simulink model "Regler_Block"  (Simulink 7.5)
settings: Solver=ode45  StartTime=0.0  StopTime=10.0  RelTol=1e-3
values from neighbouring files (symbols this model uses):
  K_ret = place(System.a, System.b, [-18 -10 -9 -5 -7])    [Test_Reglerauslegung.m]    (also in auslegung.m = place(System.a, System.b, [-2 -4 -3]))
  KV = KV'    [Reglerauslegung.m]    (also in Test_Reglerauslegung.m; auslegung.m)
undefined symbols (not defined in the file or in its folder): Control_lib, PID_Regler, Ts
libraries: simulink x8
settings Model: Creator=Mattse  LastModifiedBy=Mattse

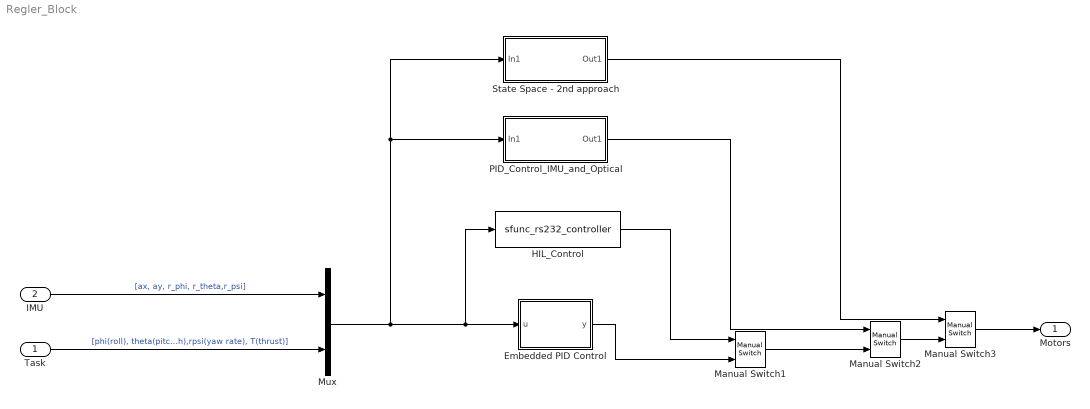
== system Regler_Block ==
  Task : Inport  PortDimensions=4  DataType=double  OutDataTypeStr=double
  IMU : Inport  Port=2
  Embedded PID Control : Stateflow chart  TreatAsAtomicUnit=on
  HIL_Control : S-Function  FunctionName=sfunc_rs232_controller  Parameters=Config  EnableBusSupport=off  mask{enabled=off}
      mask prompts: enabled "Enable this Block:"
      mask init:
      | Config.Enabled = enabled;
  Manual Switch1 : simulink/Signal Routing/Manual Switch  SystemSampleTime=-1  sw=1  action=0  varsize=off
  Manual Switch2 : simulink/Signal Routing/Manual Switch  SystemSampleTime=-1  sw=0  action=0  varsize=off
  Manual Switch3 : simulink/Signal Routing/Manual Switch  SystemSampleTime=-1  sw=1  action=0  varsize=off
  Mux : Mux  Inputs=2
  PID_Control_IMU_and_Optical : Subsystem  AncestorBlock=Control_lib/PID_Regler
  State Space - 2nd approach : Subsystem
  Motors : Outport  PortDimensions=4
  wires:
  IMU/1 -> Mux/1  "[ax, ay, r_phi, r_theta,r_psi]"
  Task/1 -> Mux/2  "[phi(roll), theta(pitch),rpsi(yaw rate), T(thrust)]"
  Mux/1 -> PID_Control_IMU_and_Optical/1(In1), State Space - 2nd approach/1(In1), HIL_Control/1, Embedded PID Control/1(u)
  Manual Switch1/1 -> Manual Switch2/2
  Embedded PID Control/1(y) -> Manual Switch1/2
  HIL_Control/1 -> Manual Switch1/1
  PID_Control_IMU_and_Optical/1(Out1) -> Manual Switch2/1
  Manual Switch2/1 -> Manual Switch3/2
  Manual Switch3/1 -> Motors/1
  State Space - 2nd approach/1(Out1) -> Manual Switch3/1

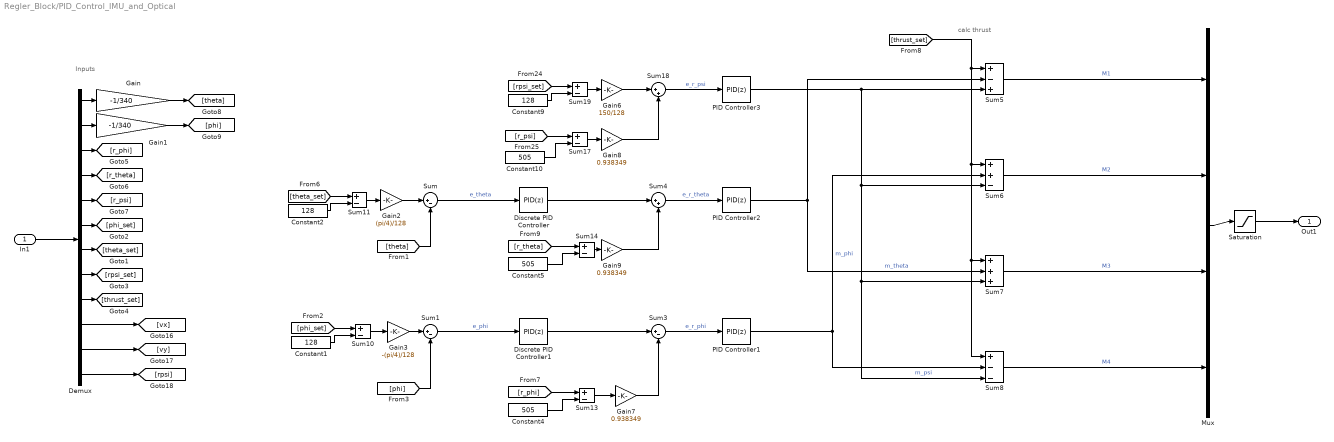
== system Regler_Block/PID_Control_IMU_and_Optical ==
  note: calc thrust
  note: Inputs
  In1 : Inport  OutDataType=fixdt(1, 16)  OutScaling=2^0
  Constant1 : Constant  Value=128  OutDataType=fixdt(1, 16)  OutScaling=2^0
  Constant10 : Constant  Value=505  OutDataType=fixdt(1, 16)  OutScaling=2^0
  Constant2 : Constant  Value=128  OutDataType=fixdt(1, 16)  OutScaling=2^0
  Constant4 : Constant  Value=505  OutDataType=fixdt(1, 16)  OutScaling=2^0
  Constant5 : Constant  Value=505  OutDataType=fixdt(1, 16)  OutScaling=2^0
  Constant9 : Constant  Value=128  OutDataType=fixdt(1, 16)  OutScaling=2^0
  Demux : Demux  Outputs=12
  Discrete PID Controller : simulink/Continuous/PID Controller  DialogController=pidpack.PIDConfig.pidDDGCreate  DialogControllerArgs=DataTag0  SystemSampleTime=-1  Controller=PID  TimeDomain=Discrete-time  SampleTime=Ts  IntegratorMethod=Forward Euler  FilterMethod=Forward Euler  Form=Ideal  P=150  I=0.5  D=0  N=0  InitialConditionSource=internal  InitialConditionForIntegrator=0  InitialConditionForFilter=0  ExternalReset=none  ZeroCross=off  LimitOutput=off  UpperSaturationLimit=inf  LowerSaturationLimit=-inf  LinearizeAsGain=off  AntiWindupMode=none  Kb=1  TrackingMode=off  Kt=1  PParamMin=[]  PParamMax=[]  IParamMin=[]  IParamMax=[]  DParamMin=[]  DParamMax=[]  NParamMin=[]  NParamMax=[]  KbParamMin=[]  KbParamMax=[]  KtParamMin=[]  KtParamMax=[]  POutMin=[]  POutMax=[]  IOutMin=[]  IOutMax=[]  DOutMin=[]  DOutMax=[]  NOutMin=[]  NOutMax=[]  KbOutMin=[]  KbOutMax=[]  KtOutMin=[]  KtOutMax=[]  IntegratorOutMin=[]  IntegratorOutMax=[]  FilterOutMin=[]  FilterOutMax=[]  SumOutMin=[]  SumOutMax=[]  SumI1OutMin=[]  SumI1OutMax=[]  SumI2OutMin=[]  SumI2OutMax=[]  SumI3OutMin=[]  SumI3OutMax=[]  SumDOutMin=[]  SumDOutMax=[]  SaturationOutMin=[]  SaturationOutMax=[]  IntegratorContinuousStateAttributes=''  IntegratorStateMustResolveToSignalObject=off  IntegratorRTWStateStorageClass=Auto  FilterContinuousStateAttributes=''  FilterStateMustResolveToSignalObject=off  FilterRTWStateStorageClass=Auto
  Discrete PID Controller1 : simulink/Continuous/PID Controller  DialogController=pidpack.PIDConfig.pidDDGCreate  DialogControllerArgs=DataTag1  SystemSampleTime=-1  Controller=PID  TimeDomain=Discrete-time  SampleTime=Ts  IntegratorMethod=Forward Euler  FilterMethod=Forward Euler  Form=Ideal  P=150  I=0.5  D=0  N=0  InitialConditionSource=internal  InitialConditionForIntegrator=0  InitialConditionForFilter=0  ExternalReset=none  ZeroCross=off  LimitOutput=off  UpperSaturationLimit=inf  LowerSaturationLimit=-inf  LinearizeAsGain=off  AntiWindupMode=none  Kb=1  TrackingMode=off  Kt=1  PParamMin=[]  PParamMax=[]  IParamMin=[]  IParamMax=[]  DParamMin=[]  DParamMax=[]  NParamMin=[]  NParamMax=[]  KbParamMin=[]  KbParamMax=[]  KtParamMin=[]  KtParamMax=[]  POutMin=[]  POutMax=[]  IOutMin=[]  IOutMax=[]  DOutMin=[]  DOutMax=[]  NOutMin=[]  NOutMax=[]  KbOutMin=[]  KbOutMax=[]  KtOutMin=[]  KtOutMax=[]  IntegratorOutMin=[]  IntegratorOutMax=[]  FilterOutMin=[]  FilterOutMax=[]  SumOutMin=[]  SumOutMax=[]  SumI1OutMin=[]  SumI1OutMax=[]  SumI2OutMin=[]  SumI2OutMax=[]  SumI3OutMin=[]  SumI3OutMax=[]  SumDOutMin=[]  SumDOutMax=[]  SaturationOutMin=[]  SaturationOutMax=[]  IntegratorContinuousStateAttributes=''  IntegratorStateMustResolveToSignalObject=off  IntegratorRTWStateStorageClass=Auto  FilterContinuousStateAttributes=''  FilterStateMustResolveToSignalObject=off  FilterRTWStateStorageClass=Auto
  Gain : Gain  Gain=-1/340  ParameterDataType=fixdt(1, 16)  ParameterScaling=2^0  OutDataType=fixdt(1, 16)  OutScaling=2^0
  Gain1 : Gain  Gain=-1/340  ParameterDataType=fixdt(1, 16)  ParameterScaling=2^0  OutDataType=fixdt(1, 16)  OutScaling=2^0
  Gain2 : Gain  Gain=(pi/4)/128  ParameterDataType=fixdt(1, 16)  ParameterScaling=2^0  OutDataType=fixdt(1, 16)  OutScaling=2^0
  Gain3 : Gain  Gain=-(pi/4)/128  ParameterDataType=fixdt(1, 16)  ParameterScaling=2^0  OutDataType=fixdt(1, 16)  OutScaling=2^0
  Gain6 : Gain  Gain=150/128  ParameterDataType=fixdt(1, 16)  ParameterScaling=2^0  OutDataType=fixdt(1, 16)  OutScaling=2^0
  Gain7 : Gain  Gain=0.938349  ParameterDataType=fixdt(1, 16)  ParameterScaling=2^0  OutDataType=fixdt(1, 16)  OutScaling=2^0
  Gain8 : Gain  Gain=0.938349  ParameterDataType=fixdt(1, 16)  ParameterScaling=2^0  OutDataType=fixdt(1, 16)  OutScaling=2^0
  Gain9 : Gain  Gain=0.938349  ParameterDataType=fixdt(1, 16)  ParameterScaling=2^0  OutDataType=fixdt(1, 16)  OutScaling=2^0
  Mux : Mux
  PID Controller1 : simulink/Continuous/PID Controller  DialogController=pidpack.PIDConfig.pidDDGCreate  DialogControllerArgs=DataTag2  SystemSampleTime=-1  Controller=PID  TimeDomain=Discrete-time  SampleTime=Ts  IntegratorMethod=Forward Euler  FilterMethod=Forward Euler  Form=Ideal  P=60  I=0.5  D=0  N=0  InitialConditionSource=internal  InitialConditionForIntegrator=0  InitialConditionForFilter=0  ExternalReset=none  ZeroCross=off  LimitOutput=off  UpperSaturationLimit=inf  LowerSaturationLimit=-inf  LinearizeAsGain=off  AntiWindupMode=none  Kb=1  TrackingMode=off  Kt=1  PParamMin=[]  PParamMax=[]  IParamMin=[]  IParamMax=[]  DParamMin=[]  DParamMax=[]  NParamMin=[]  NParamMax=[]  KbParamMin=[]  KbParamMax=[]  KtParamMin=[]  KtParamMax=[]  POutMin=[]  POutMax=[]  IOutMin=[]  IOutMax=[]  DOutMin=[]  DOutMax=[]  NOutMin=[]  NOutMax=[]  KbOutMin=[]  KbOutMax=[]  KtOutMin=[]  KtOutMax=[]  IntegratorOutMin=[]  IntegratorOutMax=[]  FilterOutMin=[]  FilterOutMax=[]  SumOutMin=[]  SumOutMax=[]  SumI1OutMin=[]  SumI1OutMax=[]  SumI2OutMin=[]  SumI2OutMax=[]  SumI3OutMin=[]  SumI3OutMax=[]  SumDOutMin=[]  SumDOutMax=[]  SaturationOutMin=[]  SaturationOutMax=[]  IntegratorContinuousStateAttributes=''  IntegratorStateMustResolveToSignalObject=off  IntegratorRTWStateStorageClass=Auto  FilterContinuousStateAttributes=''  FilterStateMustResolveToSignalObject=off  FilterRTWStateStorageClass=Auto
  PID Controller2 : simulink/Continuous/PID Controller  DialogController=pidpack.PIDConfig.pidDDGCreate  DialogControllerArgs=DataTag3  SystemSampleTime=-1  Controller=PID  TimeDomain=Discrete-time  SampleTime=Ts  IntegratorMethod=Forward Euler  FilterMethod=Forward Euler  Form=Ideal  P=60  I=0.5  D=0  N=0  InitialConditionSource=internal  InitialConditionForIntegrator=0  InitialConditionForFilter=0  ExternalReset=none  ZeroCross=off  LimitOutput=off  UpperSaturationLimit=inf  LowerSaturationLimit=-inf  LinearizeAsGain=off  AntiWindupMode=none  Kb=1  TrackingMode=off  Kt=1  PParamMin=[]  PParamMax=[]  IParamMin=[]  IParamMax=[]  DParamMin=[]  DParamMax=[]  NParamMin=[]  NParamMax=[]  KbParamMin=[]  KbParamMax=[]  KtParamMin=[]  KtParamMax=[]  POutMin=[]  POutMax=[]  IOutMin=[]  IOutMax=[]  DOutMin=[]  DOutMax=[]  NOutMin=[]  NOutMax=[]  KbOutMin=[]  KbOutMax=[]  KtOutMin=[]  KtOutMax=[]  IntegratorOutMin=[]  IntegratorOutMax=[]  FilterOutMin=[]  FilterOutMax=[]  SumOutMin=[]  SumOutMax=[]  SumI1OutMin=[]  SumI1OutMax=[]  SumI2OutMin=[]  SumI2OutMax=[]  SumI3OutMin=[]  SumI3OutMax=[]  SumDOutMin=[]  SumDOutMax=[]  SaturationOutMin=[]  SaturationOutMax=[]  IntegratorContinuousStateAttributes=''  IntegratorStateMustResolveToSignalObject=off  IntegratorRTWStateStorageClass=Auto  FilterContinuousStateAttributes=''  FilterStateMustResolveToSignalObject=off  FilterRTWStateStorageClass=Auto
  PID Controller3 : simulink/Continuous/PID Controller  DialogController=pidpack.PIDConfig.pidDDGCreate  DialogControllerArgs=DataTag4  SystemSampleTime=-1  Controller=PID  TimeDomain=Discrete-time  SampleTime=Ts  IntegratorMethod=Forward Euler  FilterMethod=Forward Euler  Form=Ideal  P=60  I=0.5  D=0  N=0  InitialConditionSource=internal  InitialConditionForIntegrator=0  InitialConditionForFilter=0  ExternalReset=none  ZeroCross=off  LimitOutput=off  UpperSaturationLimit=inf  LowerSaturationLimit=-inf  LinearizeAsGain=off  AntiWindupMode=none  Kb=1  TrackingMode=off  Kt=1  PParamMin=[]  PParamMax=[]  IParamMin=[]  IParamMax=[]  DParamMin=[]  DParamMax=[]  NParamMin=[]  NParamMax=[]  KbParamMin=[]  KbParamMax=[]  KtParamMin=[]  KtParamMax=[]  POutMin=[]  POutMax=[]  IOutMin=[]  IOutMax=[]  DOutMin=[]  DOutMax=[]  NOutMin=[]  NOutMax=[]  KbOutMin=[]  KbOutMax=[]  KtOutMin=[]  KtOutMax=[]  IntegratorOutMin=[]  IntegratorOutMax=[]  FilterOutMin=[]  FilterOutMax=[]  SumOutMin=[]  SumOutMax=[]  SumI1OutMin=[]  SumI1OutMax=[]  SumI2OutMin=[]  SumI2OutMax=[]  SumI3OutMin=[]  SumI3OutMax=[]  SumDOutMin=[]  SumDOutMax=[]  SaturationOutMin=[]  SaturationOutMax=[]  IntegratorContinuousStateAttributes=''  IntegratorStateMustResolveToSignalObject=off  IntegratorRTWStateStorageClass=Auto  FilterContinuousStateAttributes=''  FilterStateMustResolveToSignalObject=off  FilterRTWStateStorageClass=Auto
  Saturation : Saturate  UpperLimit=255  LowerLimit=0  OutDataType=fixdt(1, 16)  OutScaling=2^0
  Sum : Sum  Inputs=|+-  OutDataType=fixdt(1, 16)  OutScaling=2^0
  Sum1 : Sum  Inputs=|+-  OutDataType=fixdt(1, 16)  OutScaling=2^0
  Sum{10..11,13..14,17,19} (6 alike) : Sum  Inputs=+-  OutDataType=fixdt(1, 16)  OutScaling=2^0
  Sum18 : Sum  Inputs=|++  OutDataType=fixdt(1, 16)  OutScaling=2^0
  Sum3 : Sum  Inputs=|+-  OutDataType=fixdt(1, 16)  OutScaling=2^0
  Sum4 : Sum  Inputs=|++  OutDataType=fixdt(1, 16)  OutScaling=2^0
  Sum5 : Sum  Inputs=+-+  OutDataType=fixdt(1, 16)  OutScaling=2^0
  Sum6 : Sum  Inputs=++-  OutDataType=fixdt(1, 16)  OutScaling=2^0
  Sum7 : Sum  Inputs=+++  OutDataType=fixdt(1, 16)  OutScaling=2^0
  Sum8 : Sum  Inputs=+--  OutDataType=fixdt(1, 16)  OutScaling=2^0
  Out1 : Outport  OutDataType=fixdt(1, 16)  OutScaling=2^0
  wires:
  Sum14/1 -> Gain9/1
  Gain9/1 -> Sum4/2
  Sum13/1 -> Gain7/1
  Gain3/1 -> Sum1/1
  Gain2/1 -> Sum/1
  Sum11/1 -> Gain2/1
  Sum10/1 -> Gain3/1
  [r_theta] -> Sum14/1
  Constant5/1 -> Sum14/2
  [r_phi] -> Sum13/1
  Constant4/1 -> Sum13/2
  Constant2/1 -> Sum11/2
  [theta_set] -> Sum11/1
  Constant1/1 -> Sum10/2
  [phi_set] -> Sum10/1
  Saturation/1 -> Out1/1
  Mux/1 -> Saturation/1
  [thrust_set] -> Sum8/1, Sum7/1, Sum6/1, Sum5/1
  PID Controller1/1 -> Sum6/2, Sum8/2  "m_phi"
  Sum6/1 -> Mux/2  "M2"
  Sum7/1 -> Mux/3  "M3"
  Sum8/1 -> Mux/4  "M4"
  Sum5/1 -> Mux/1  "M1"
  Sum4/1 -> PID Controller2/1  "e_r_theta"
  Sum3/1 -> PID Controller1/1  "e_r_phi"
  Sum1/1 -> Discrete PID Controller1/1  "e_phi"
  [phi] -> Sum1/2
  Sum/1 -> Discrete PID Controller/1  "e_theta"
  [theta] -> Sum/2
  Gain1/1 -> [phi]
  Gain/1 -> [theta]
  Demux/9 -> [thrust_set]
  Demux/8 -> [rpsi_set]
  Demux/7 -> [theta_set]
  Demux/6 -> [phi_set]
  Demux/5 -> [r_psi]
  Demux/4 -> [r_theta]
  Demux/3 -> [r_phi]
  Demux/1 -> Gain/1
  Demux/2 -> Gain1/1
  In1/1 -> Demux/1
  Demux/10 -> [vx]
  Demux/11 -> [vy]
  Demux/12 -> [rpsi]
  Gain8/1 -> Sum18/2
  Sum17/1 -> Gain8/1
  Gain6/1 -> Sum18/1
  Sum19/1 -> Gain6/1
  Constant10/1 -> Sum17/2
  [r_psi] -> Sum17/1
  Constant9/1 -> Sum19/2
  [rpsi_set] -> Sum19/1
  Sum18/1 -> PID Controller3/1  "e_r_psi"
  Discrete PID Controller1/1 -> Sum3/1
  Discrete PID Controller/1 -> Sum4/1
  Gain7/1 -> Sum3/2
  PID Controller3/1 -> Sum5/3, Sum6/3, Sum7/3, Sum8/3  "m_psi"
  PID Controller2/1 -> Sum7/2, Sum5/2  "m_theta"

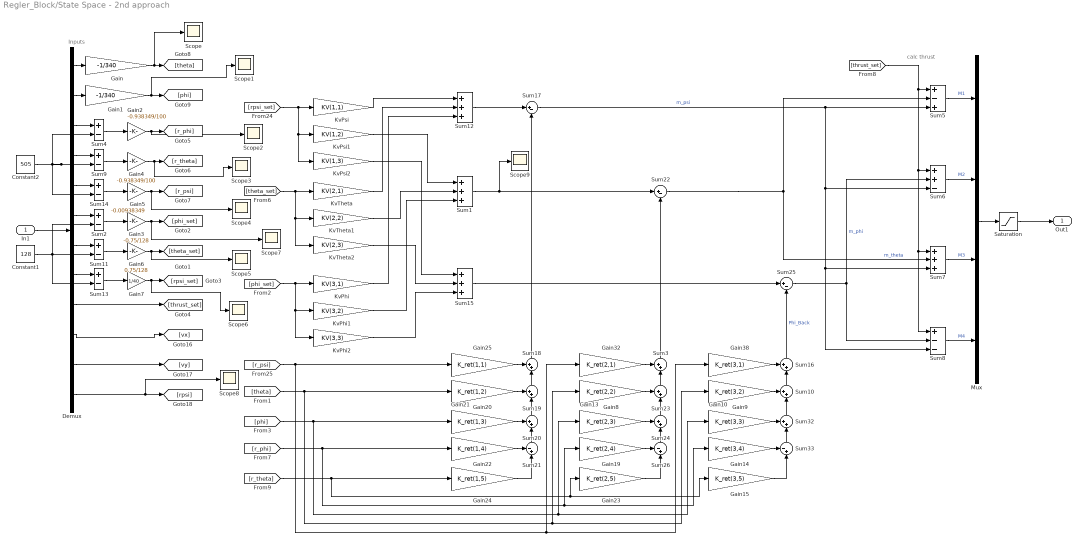
== system Regler_Block/State Space - 2nd approach ==
  note: calc thrust
  note: Inputs
  In1 : Inport  OutDataType=fixdt(1, 16)  OutScaling=2^0
  Constant1 : Constant  Value=128  OutDataType=fixdt(1, 16)  OutScaling=2^0
  Constant2 : Constant  Value=505  OutDataType=fixdt(1, 16)  OutScaling=2^0
  Demux : Demux  Outputs=12
  Gain : Gain  Gain=-1/340  ParameterDataType=fixdt(1, 16)  ParameterScaling=2^0  OutDataType=fixdt(1, 16)  OutScaling=2^0
  Gain1 : Gain  Gain=-1/340  ParameterDataType=fixdt(1, 16)  ParameterScaling=2^0  OutDataType=fixdt(1, 16)  OutScaling=2^0
  Gain10 : Gain  Gain=K_ret(3,3)  ParameterDataType=fixdt(1, 16)  ParameterScaling=2^0  OutDataType=fixdt(1, 16)  OutScaling=2^0
  Gain13 : Gain  Gain=K_ret(2,3)  ParameterDataType=fixdt(1, 16)  ParameterScaling=2^0  OutDataType=fixdt(1, 16)  OutScaling=2^0
  Gain14 : Gain  Gain=K_ret(3,4)  ParameterDataType=fixdt(1, 16)  ParameterScaling=2^0  OutDataType=fixdt(1, 16)  OutScaling=2^0
  Gain15 : Gain  Gain=K_ret(3,5)  ParameterDataType=fixdt(1, 16)  ParameterScaling=2^0  OutDataType=fixdt(1, 16)  OutScaling=2^0
  Gain19 : Gain  Gain=K_ret(2,4)  ParameterDataType=fixdt(1, 16)  ParameterScaling=2^0  OutDataType=fixdt(1, 16)  OutScaling=2^0
  Gain2 : Gain  Gain=-0.938349/100  ParameterDataType=fixdt(1, 16)  ParameterScaling=2^0  OutDataType=fixdt(1, 16)  OutScaling=2^0
  Gain20 : Gain  Gain=K_ret(1,2)  ParameterDataType=fixdt(1, 16)  ParameterScaling=2^0  OutDataType=fixdt(1, 16)  OutScaling=2^0
  Gain21 : Gain  Gain=K_ret(1,3)  ParameterDataType=fixdt(1, 16)  ParameterScaling=2^0  OutDataType=fixdt(1, 16)  OutScaling=2^0
  Gain22 : Gain  Gain=K_ret(1,4)  ParameterDataType=fixdt(1, 16)  ParameterScaling=2^0  OutDataType=fixdt(1, 16)  OutScaling=2^0
  Gain23 : Gain  Gain=K_ret(2,5)  ParameterDataType=fixdt(1, 16)  ParameterScaling=2^0  OutDataType=fixdt(1, 16)  OutScaling=2^0
  Gain24 : Gain  Gain=K_ret(1,5)  ParameterDataType=fixdt(1, 16)  ParameterScaling=2^0  OutDataType=fixdt(1, 16)  OutScaling=2^0
  Gain25 : Gain  Gain=K_ret(1,1)  ParameterDataType=fixdt(1, 16)  ParameterScaling=2^0  OutDataType=fixdt(1, 16)  OutScaling=2^0
  Gain3 : Gain  Gain=-0.75/128  ParameterDataType=fixdt(1, 16)  ParameterScaling=2^0  OutDataType=fixdt(1, 16)  OutScaling=2^0
  Gain32 : Gain  Gain=K_ret(2,1)  ParameterDataType=fixdt(1, 16)  ParameterScaling=2^0  OutDataType=fixdt(1, 16)  OutScaling=2^0
  Gain38 : Gain  Gain=K_ret(3,1)  ParameterDataType=fixdt(1, 16)  ParameterScaling=2^0  OutDataType=fixdt(1, 16)  OutScaling=2^0
  Gain4 : Gain  Gain=-0.938349/100  ParameterDataType=fixdt(1, 16)  ParameterScaling=2^0  OutDataType=fixdt(1, 16)  OutScaling=2^0
  Gain5 : Gain  Gain=-0.00938349  ParameterDataType=fixdt(1, 16)  ParameterScaling=2^0  OutDataType=fixdt(1, 16)  OutScaling=2^0
  Gain6 : Gain  Gain=0.75/128  ParameterDataType=fixdt(1, 16)  ParameterScaling=2^0  OutDataType=fixdt(1, 16)  OutScaling=2^0
  Gain7 : Gain  Gain=1/40  ParameterDataType=fixdt(1, 16)  ParameterScaling=2^0  OutDataType=fixdt(1, 16)  OutScaling=2^0
  Gain8 : Gain  Gain=K_ret(2,2)  ParameterDataType=fixdt(1, 16)  ParameterScaling=2^0  OutDataType=fixdt(1, 16)  OutScaling=2^0
  Gain9 : Gain  Gain=K_ret(3,2)  ParameterDataType=fixdt(1, 16)  ParameterScaling=2^0  OutDataType=fixdt(1, 16)  OutScaling=2^0
  KvPhi : Gain  Gain=KV(3,1)  ParameterDataType=fixdt(1, 16)  ParameterScaling=2^0  OutDataType=fixdt(1, 16)  OutScaling=2^0
  KvPhi1 : Gain  Gain=KV(3,2)  ParameterDataType=fixdt(1, 16)  ParameterScaling=2^0  OutDataType=fixdt(1, 16)  OutScaling=2^0
  KvPhi2 : Gain  Gain=KV(3,3)  ParameterDataType=fixdt(1, 16)  ParameterScaling=2^0  OutDataType=fixdt(1, 16)  OutScaling=2^0
  KvPsi : Gain  Gain=KV(1,1)  ParameterDataType=fixdt(1, 16)  ParameterScaling=2^0  OutDataType=fixdt(1, 16)  OutScaling=2^0
  KvPsi1 : Gain  Gain=KV(1,2)  ParameterDataType=fixdt(1, 16)  ParameterScaling=2^0  OutDataType=fixdt(1, 16)  OutScaling=2^0
  KvPsi2 : Gain  Gain=KV(1,3)  ParameterDataType=fixdt(1, 16)  ParameterScaling=2^0  OutDataType=fixdt(1, 16)  OutScaling=2^0
  KvTheta : Gain  Gain=KV(2,1)  ParameterDataType=fixdt(1, 16)  ParameterScaling=2^0  OutDataType=fixdt(1, 16)  OutScaling=2^0
  KvTheta1 : Gain  Gain=KV(2,2)  ParameterDataType=fixdt(1, 16)  ParameterScaling=2^0  OutDataType=fixdt(1, 16)  OutScaling=2^0
  KvTheta2 : Gain  Gain=KV(2,3)  ParameterDataType=fixdt(1, 16)  ParameterScaling=2^0  OutDataType=fixdt(1, 16)  OutScaling=2^0
  Mux : Mux
  Saturation : Saturate  UpperLimit=255  LowerLimit=0  OutDataType=fixdt(1, 16)  OutScaling=2^0
  Scope{,1..9} (10 alike) : Scope
      Scope settings: SaveName=ScopeData17
      Scope1 settings: SaveName=ScopeData20
      Scope2 settings: SaveName=ScopeData21
      Scope3 settings: SaveName=ScopeData22
      Scope4 settings: SaveName=ScopeData23
      Scope5 settings: SaveName=ScopeData24
      Scope6 settings: SaveName=ScopeData25
      Scope7 settings: SaveName=ScopeData26
      Scope8 settings: SaveName=ScopeData27
      Scope9 settings: SaveName=ScopeData28
  Sum{1,7,12,15} (4 alike) : Sum  Inputs=+++  OutDataType=fixdt(1, 16)  OutScaling=2^0
  Sum{3,10,16,18..20,23..24,32} (9 alike) : Sum  Inputs=++|  OutDataType=fixdt(1, 16)  OutScaling=2^0
  Sum{2,4,9,11,13..14} (6 alike) : Sum  Inputs=+-  OutDataType=fixdt(1, 16)  OutScaling=2^0
  Sum17 : Sum  Inputs=|+-  OutDataType=fixdt(1, 16)  OutScaling=2^0
  Sum21 : Sum  Inputs=-+|  OutDataType=fixdt(1, 16)  OutScaling=2^0
  Sum22 : Sum  Inputs=|+-  OutDataType=fixdt(1, 16)  OutScaling=2^0
  Sum25 : Sum  Inputs=|+-  OutDataType=fixdt(1, 16)  OutScaling=2^0
  Sum26 : Sum  Inputs=-+|  OutDataType=fixdt(1, 16)  OutScaling=2^0
  Sum33 : Sum  Inputs=-+|  OutDataType=fixdt(1, 16)  OutScaling=2^0
  Sum5 : Sum  Inputs=+-+  OutDataType=fixdt(1, 16)  OutScaling=2^0
  Sum6 : Sum  Inputs=++-  OutDataType=fixdt(1, 16)  OutScaling=2^0
  Sum8 : Sum  Inputs=+--  OutDataType=fixdt(1, 16)  OutScaling=2^0
  Out1 : Outport  OutDataType=fixdt(1, 16)  OutScaling=2^0
  wires:
  Saturation/1 -> Out1/1
  Mux/1 -> Saturation/1
  [thrust_set] -> Sum8/1, Sum7/1, Sum6/1, Sum5/1
  Sum25/1 -> Sum6/2, Sum8/2  "m_phi"
  Sum6/1 -> Mux/2  "M2"
  Sum7/1 -> Mux/3  "M3"
  Sum8/1 -> Mux/4  "M4"
  Sum5/1 -> Mux/1  "M1"
  Gain1/1 -> [phi], Scope1/1
  Gain/1 -> [theta], Scope/1
  Demux/9 -> [thrust_set]
  Demux/1 -> Gain/1
  Demux/2 -> Gain1/1
  In1/1 -> Demux/1
  Demux/10 -> [vx]
  Demux/11 -> [vy]
  Demux/12 -> [rpsi], Scope8/1
  Sum17/1 -> Sum5/3, Sum6/3, Sum7/3, Sum8/3  "m_psi"
  [phi_set] -> KvPhi/1, KvPhi1/1, KvPhi2/1
  [rpsi_set] -> KvPsi/1, KvPsi2/1, KvPsi1/1
  Demux/3 -> Sum4/1
  Sum4/1 -> Gain2/1
  Constant2/1 -> Sum4/2, Sum9/2, Sum14/2
  Gain2/1 -> [r_phi], Scope2/1
  Demux/4 -> Sum9/1
  Sum9/1 -> Gain4/1
  Gain4/1 -> [r_theta], Scope3/1
  Gain5/1 -> [r_psi], Scope4/1
  Demux/5 -> Sum14/1
  Sum14/1 -> Gain5/1
  KvPsi/1 -> Sum12/1
  KvTheta/1 -> Sum12/2
  KvPhi/1 -> Sum12/3
  KvPsi1/1 -> Sum1/1
  KvTheta1/1 -> Sum1/2
  KvPhi1/1 -> Sum1/3
  KvPhi2/1 -> Sum15/3
  KvTheta2/1 -> Sum15/2
  KvPsi2/1 -> Sum15/1
  [theta_set] -> KvTheta/1, KvTheta1/1, KvTheta2/1
  Gain3/1 -> [phi_set], Scope7/1
  Demux/6 -> Sum2/1
  Sum2/1 -> Gain3/1
  Constant1/1 -> Sum2/2, Sum13/2, Sum11/2
  Gain7/1 -> [rpsi_set], Scope6/1
  Gain6/1 -> [theta_set], Scope5/1
  Sum11/1 -> Gain6/1
  Sum13/1 -> Gain7/1
  Demux/8 -> Sum13/1
  Demux/7 -> Sum11/1
  Gain8/1 -> Sum23/1
  Sum24/1 -> Sum23/2
  Sum23/1 -> Sum3/2
  Sum26/1 -> Sum24/2
  Gain23/1 -> Sum26/2
  Sum32/1 -> Sum10/2
  Sum10/1 -> Sum16/2
  Sum33/1 -> Sum32/2
  Gain19/1 -> Sum26/1
  Gain13/1 -> Sum24/1
  Gain32/1 -> Sum3/1
  Gain38/1 -> Sum16/1
  Gain9/1 -> Sum10/1
  Gain10/1 -> Sum32/1
  Gain14/1 -> Sum33/1
  Gain15/1 -> Sum33/2
  Gain25/1 -> Sum18/1
  Sum20/1 -> Sum19/2
  Sum19/1 -> Sum18/2
  Sum21/1 -> Sum20/2
  Gain24/1 -> Sum21/2
  Gain22/1 -> Sum21/1
  Gain21/1 -> Sum20/1
  Gain20/1 -> Sum19/1
  [r_psi] -> Gain25/1, Gain32/1, Gain38/1
  [theta] -> Gain20/1, Gain8/1, Gain9/1
  [phi] -> Gain21/1, Gain13/1, Gain10/1
  [r_phi] -> Gain22/1, Gain19/1, Gain14/1
  [r_theta] -> Gain24/1, Gain23/1, Gain15/1
  Sum12/1 -> Sum17/1
  Sum18/1 -> Sum17/2
  Sum1/1 -> Sum22/1, Scope9/1
  Sum3/1 -> Sum22/2
  Sum22/1 -> Sum7/2, Sum5/2  "m_theta"
  Sum16/1 -> Sum25/2  "Phi_Back"
  Sum15/1 -> Sum25/1

== matlab function Embedded PID Control ==
  settings: updateMethod=DISCRETE  sampleTime=0.005
  data: u input double; y output double
function y = fcn(u)
%#eml
persistent e_r_Roll_1 e_Roll_1 r_Roll_I_State r_Roll_Filter_State 
persistent e_r_Pitch_1 e_Pitch_1 r_Pitch_I_State r_Pitch_Filter_State 
persistent e_r_Yaw_1 r_Yaw_I_State r_Yaw_Filter_State
persistent M1_limited M2_limited M3_limited M4_limited 
%  first time initialization
if isempty(M1_limited) 
    M1_limited=uint8(0);
    M2_limited=uint8(0);
    M3_limited=uint8(0);
    M4_limited=uint8(0);
    e_r_Roll_1 = double(0);
    e_Roll_1 = double(0);
    r_Roll_I_State = double(0);
    r_Roll_Filter_State = double(0); 
    e_r_Pitch_1 = double(0);
    e_Pitch_1 = double(0);
    r_Pitch_I_State = double(0); 
    r_Pitch_Filter_State = double(0); 
    e_r_Yaw_1 = double(0); 
    r_Yaw_I_State = double(0); 
    r_Yaw_Filter_State = double(0);
end
IRoll = double(0);
FiltRoll = double(0);
IPitch = double(0);
FiltPitch = double(0);
Ts = 0.005; % sec
G = 9.810; % m/sec²
maxRemotePitch = 128;
maxRemoteRoll = 128;
maxRemoteYaw = 128;
maxPitchAngle = pi/4;
maxRollAngle  = pi/4;
maxYawRate = 200;
sensorSensitivityX = 340;
sensorSensitivityY = 340;
sensorSensitivityZ = 340;
copterState.gyroPOffset = 505;
copterState.gyroROffset = 505;
copterState.gyroYOffset = 505;
copterState.YawRateI_State = 0;
copterState.YawRateD_Filter = 0;
copterState.PitchRateI_State = 0;
copterState.PitchRateD_Filter = 0;
copterState.RollRateI_State = 0;
copterState.RollRateD_Filter = 0;
% copy inputs to variables with easy to know names
copterState.angVelRRaw =  u(3);
copterState.accYRaw = u(2);
copterState.angVelPRaw = u(4);
copterState.accXRaw = u(1);
copterState.accZRaw = 0; %not available
copterState.angVelYRaw = u(5);
copterState.remoteForceRaw = u(9);
copterState.remotePitchRaw = u(7);
copterState.remoteRollRaw = u(6);
copterState.remoteYawRaw = u(8);
copterState.accY = int16(0);
copterState.accX = int16(0);
copterState.accZ = int16(0);
copterState.angP = int16(0);
copterState.angR = int16(0);
copterState.angVelP = int16(0);
copterState.angVelR = int16(0);
copterState.angVelY = int16(0);
copterState.remotePitch = int16(0);
copterState.remoteRoll = int16(0);
copterState.remoteForce = int16(0);
copterState.remoteYaw = int16(0);
angP = double(0);
angR = double(0);

% Convert Data like in the copter
% Accelerometer
%%%%%%%%%%%%%%%%%
  %/* calculate the physical acceleration values in [(10 * m)/(s^2)], as needed by the control algorithm */
  copterState.accY = int16(((int32(copterState.accYRaw) * G) / sensorSensitivityY) / 10);
  copterState.accX = -int16(((int32(copterState.accXRaw) * G) / sensorSensitivityX) / 10);
  copterState.accZ = -int16(((int32(copterState.accZRaw) * G) / sensorSensitivityZ) / 10);
  %// [ 10000*rad ]
  copterState.angP = -int16(int32(copterState.accXRaw)*1000/340);
  copterState.angR = -int16(int32(copterState.accYRaw)*1000/340);
  
  % Gyroscopes [100 * rad/sec]
  %%%%%%%%%%%%%%
   copterState.angVelP     = -int16(double(copterState.angVelPRaw-copterState.gyroPOffset) * 0.938349);
   copterState.angVelR     = int16(double(copterState.angVelRRaw-copterState.gyroROffset) * 0.938349);
   copterState.angVelY     = -int16(double(copterState.angVelYRaw-copterState.gyroYOffset) * 0.938349);
   
   % Remote
   %%%%%%%%%%%%%
  copterState.remotePitch    = int16(maxPitchAngle*int32(copterState.remotePitchRaw-128)/maxRemotePitch);
  copterState.remoteRoll     = -int16(maxRollAngle*int32(copterState.remoteRollRaw-128)/maxRemoteRoll);
  copterState.remoteForce    = int16(copterState.remoteForceRaw); 
  copterState.remoteYaw      = int16(maxYawRate*int32(copterState.remoteYawRaw-128)/maxRemoteYaw);

% Set outputs to Values calculated last sample time
y = double([M1_limited;M2_limited;M3_limited;M4_limited]);
   
   angP = double(copterState.angP)/1000;
   angR = double(copterState.angR)/1000;
   
% calculate error values for the controlled angles
   % Pitch error 
   e_Pitch = double(copterState.remotePitch) - angP;
   % Roll error
   e_Roll = double(copterState.remoteRoll) - angR;
   % calculate controller output for the angles (I State & FilterState are not necessary cause only p is used
   [m_Roll, IRoll, FiltRoll] = PID(150,0.5,0,0,e_Roll,e_Roll_1,IRoll, FiltRoll, Ts);
   [m_Pitch, IPitch, FiltPitch] = PID(150,0.5,0,0,e_Pitch,e_Pitch_1,IPitch,FiltPitch,Ts);
      
   % Yaw Rate error
   e_r_Yaw = double(copterState.remoteYaw) - double(copterState.angVelY);
   % Pitch Rate error
   e_r_Pitch = m_Pitch - double(copterState.angVelP);
   % Roll Rate error
   e_r_Roll = m_Roll - double(copterState.angVelR);
   % calculate  controller output for rates
   [m_r_Yaw,r_Yaw_I_State, r_Yaw_Filter_State] = PID (70, ...
       0.5, 0,0,e_r_Yaw, e_r_Yaw_1, r_Yaw_I_State, r_Yaw_Filter_State,Ts);
   [m_r_Roll,r_Roll_I_State, r_Roll_Filter_State] = PID (70, ...
       0.5, 0,0,e_r_Roll, e_r_Roll_1, r_Roll_I_State, r_Roll_Filter_State,Ts);
   [m_r_Pitch,r_Pitch_I_State, r_Pitch_Filter_State] = PID (70, ...
       0.5, 0,0,e_r_Pitch, e_r_Pitch_1, r_Pitch_I_State, r_Pitch_Filter_State,Ts);
   
   % save error for next sample time
   e_Roll_1 = e_Roll;
   e_Pitch_1 = e_Pitch;
   e_r_Roll_1 = e_r_Roll;
   e_r_Pitch_1 = e_r_Pitch;
   e_r_Yaw_1 = e_r_Yaw;
 
   %//Calculate new setpoints of all motors
    M1 = (copterState.remoteForce-m_r_Pitch+m_r_Yaw);
    M2 = (copterState.remoteForce+m_r_Roll-m_r_Yaw);
    M3 = (copterState.remoteForce+m_r_Pitch+m_r_Yaw);
    M4 = (copterState.remoteForce-m_r_Roll-m_r_Yaw);
   
   
    %// saturate setpoint of motor1 to 0 if less and 255 if above
    if M1 < 0
      M1_limited = uint8(0);
    else
        if M1 > 255
            M1_limited = uint8(255); 
        else
            M1_limited=uint8(M1);
        end
    end
    
    %// saturate setpoint of motor2 to 0 if less and 255 if above
    if M2 < 0
      M2_limited = uint8(0);
    else
        if M2 > 255
          M2_limited = uint8(255); 
        else
          M2_limited=uint8(M2);
        end
    end

    %// saturate setpoint of motor3 to 0 if less and 255 if above
  if M3 < 0
      M3_limited = uint8(0);
  else
      if M3 > 255
        M3_limited = uint8(255); 
      else
         M3_limited=uint8(M3);
      end
  end
    
    %// saturate setpoint of motor4 to 0 if less and 255 if above
    if M4 < 0
      M4_limited = uint8(0);
    else
        if M4 > 255
           M4_limited = uint8(255); 
        else
           M4_limited=uint8(M4);
        end
    end

% This function calculates the next Value of the ?ideal? PID controller
function [ret, I_State, Filt_State] = PID (P, I, D, N, ek, ek_1, I_State, Filt_State, Ts)

if P ~= 0 
    if I ~= 0
        % calculate new itegral value
        I_State = ek * Ts * I + I_State;
    else
        I_State = 0;
    end

    if D ~= 0
        % calculate new derivative Value
        yd = (ek - ek_1)/Ts * D;

        % Filter the derivative  Value
        Filt_State = Ts * (yd -N*Filt_State)+ Filt_State ;
    else
        Filt_State = 0;
    end

    % Add all values and multiply P gain to all
    ret = (P * ek + I_State + Filt_State);

else
    ret = 0;
end


function ret16 = mult_fp (A, B, factor)
    ret32 = int32(A) * int32(B)/factor;
    if ret32 > 2^15-1
        ret16 = int16(2^15-1);
    else
        if ret32 < -2^15+1
            ret16 = int16(-2^15+1);
        else
            ret16 = int16(ret32);
        end
    end
% end of mult_fp    

function ret16 = div_fp(A, B, factor)
if B == 0
    display('divide by ZERO !!!!')
    ret16 = 2^16-1;
else
    ret32 = int32(A)*factor/int32(B);
     if ret32 > 2^15-1
        ret16 = int16(2^15-1);
    else
        if ret32 < -2^15+1
            ret16 = int16(-2^15+1);
        else
            ret16 = int16(ret32);
        end
    end
end
% end of div_fp
